simulink model "PMSM20180521"  (Simulink 7.9)
settings: Solver=FixedStepDiscrete  StartTime=0.0  StopTime=1  FixedStep=Auto  RelTol=1e-3
model workspace (MAT data in the model file):
  polePairs = 16
  encoderResolution = 4096
  indexOffset = 0
undefined symbols (not defined in the file or in its folder): Down, Up
libraries: idelinklib_common x37, simulink x13, c2833xlib x7, c280xlib x6, simulink_extras x2, idelinklib_ticcs x1, idelinklib_tgtpref x1
(part 1 of 3)
settings Model: Creator=ChenYu  LastModifiedBy=KING
settings DataIOCC: SaveOutput=off  SaveTime=off
settings OptimizationCC: OptimizeModelRefInitCode=on  LifeSpan=1
settings HardwareCC: ProdBitPerChar=16  ProdBitPerInt=16  ProdBitPerPointer=16  ProdLargestAtomicInteger=Integer  ProdIntDivRoundTo=Zero  ProdEndianess=LittleEndian  ProdWordSize=16  ProdHWDeviceType=Texas Instruments->C2000
settings RTWCC: SystemTargetFile=idelink_ert.tlc  GenerateMakefile=off  TemplateMakefile=none  Description=IDE Link ERT  ProcessScript=idelink_ert_make_rtw_hook
settings RTWCC: CustomInitializer=|
  | // Make sure the XINTF clock is enabled   cool
  | 	SysCtrlRegs.PCLKCR3.bit.XINTFENCLK = 1;
  | 
  | 	// Configure the GPIO for XINTF with a 16-bit data bus
  | 	// This function is in DSP2833x_Xintf.c
  | 	//InitXintf16Gpio();
  | 
  |     EALLOW;
  |     // All Zones---------------------------------
  |     // Timing for all zones based on XTIMCLK = SYSCLKOUT/2
  |     XintfRegs.XINTCNF2.bit.XTIMCLK = 1;
  |     // Buffer up to 3 writes
  |     XintfRegs.XINTCNF2.bit.WRBUFF = 3;
  |     // XCLKOUT is enabled
  |     XintfRegs.XINTCNF2.bit.CLKOFF = 0;
  |     // XCLKOUT = XTIMCLK/2
  |     XintfRegs.XINTCNF2.bit.CLKMODE = 1;
  | 
  |     // Zone 7------------------------------------
  |     // When using ready, ACTIVE must be 1 or greater
  |     // Lead must always be 1 or greater
  |     // Zone write timing
  |     XintfRegs.XTIMING7.bit.XWRLEAD = 3;//3*2*2*SYSCLKOUT
  |     XintfRegs.XTIMING7.bit.XWRACTIVE = 7; //(7+1)*2*2*SYSCLKOUT
  |     XintfRegs.XTIMING7.bit.XWRTRAIL = 3;
  |     // Zone read timing
  |     XintfRegs.XTIMING7.bit.XRDLEAD = 3;
  |     XintfRegs.XTIMING7.bit.XRDACTIVE = 7;
  |     XintfRegs.XTIMING7.bit.XRDTRAIL = 3;
  | 
  |     // double all Zone read/write lead/active/trail timing
  |     XintfRegs.XTIMING7.bit.X2TIMING = 1;
  | 
  |     // Zone will not sample XREADY signal
  |     XintfRegs.XTIMING7.bit.USEREADY = 0;
  |     XintfRegs.XTIMING7.bit.READYMODE = 0;
  | 
  |     // Size must be either:
  |     // 0,1 = x32 or
  |     // 1,1 = x16 other values are reserved
  |     XintfRegs.XTIMING7.bit.XSIZE = 3;
  | 
  |     EDIS;
  | 
  |    //Force a pipeline flush to ensure that the write to
  |    //the last register configured occurs before returning.
  |    asm(" RPT #7 || NOP");
settings CodeAppCC: IgnoreCustomStorageClasses=off
settings ERTFactory: TargetFcnLib=ansi_tfl_table_tmw.mat  CodeReplacementLibrary=ANSI_C  UtilityFuncGeneration=Auto  ERTMultiwordTypeDef=System defined  CodeExecutionProfiling=off  ERTMultiwordLength=256  MultiwordLength=2048  GenerateFullHeader=on  GenerateSampleERTMain=off  GenerateTestInterfaces=off  IsPILTarget=off  ModelReferenceCompliant=on  ParMdlRefBuildCompliant=off  CompOptLevelCompliant=off  ConcurrentExecutionCompliant=on  IncludeMdlTerminateFcn=on  GeneratePreprocessorConditionals=Disable all  CombineOutputUpdateFcns=on  CombineSignalStateStructs=off  SuppressErrorStatus=off  ERTFirstTimeCompliant=on  IncludeFileDelimiter=Auto  ERTCustomFileBanners=on  SupportAbsoluteTime=on  LogVarNameModifier=rt_  MatFileLogging=off  MultiInstanceERTCode=off  SupportNonFinite=on  SupportComplex=on  PurelyIntegerCode=off  SupportContinuousTime=off  SupportNonInlinedSFcns=off  SupportVariableSizeSignals=off  EnableShiftOperators=on  ParenthesesLevel=Nominal  PortableWordSizes=off  ModelStepFunctionPrototypeControlCompliant=on  CPPClassGenCompliant=off  AutosarCompliant=off  GRTInterface=off  GenerateErtSFunction=off  CreateSILPILBlock=None  CodeExecutionProfileVariable=executionProfile  CodeProfilingSaveOptions=SummaryOnly  GenerateASAP2=off  ExtMode=off  ExtModeTransport=0  ExtModeStaticAlloc=off  ExtModeStaticAllocSize=1000000  ExtModeTesting=off  ExtModeMexFile=TIC2000ExternalModeOpen  ExtModeIntrfLevel=Level2 - Open  InlinedParameterPlacement=Hierarchical  TargetOS=BareBoardExample  MultiInstanceErrorCode=Error  RateGroupingCode=on  RootIOFormat=Individual arguments  RTWCAPISignals=off  RTWCAPIParams=off  RTWCAPIStates=off  RTWCAPIRootIO=off  ERTSrcFileBannerTemplate=ert_code_template.cgt  ERTHdrFileBannerTemplate=ert_code_template.cgt  ERTDataSrcFileTemplate=ert_code_template.cgt  ERTDataHdrFileTemplate=ert_code_template.cgt  ERTCustomFileTemplate=example_file_process.tlc  CoverageDialogOpen=off  EnableDataOwnership=off  SignalDisplayLevel=10  ParamTuneLevel=10  GlobalDataDefinition=Auto  DataDefinitionFile=global.c  GlobalDataReference=Auto  ERTFilePackagingFormat=Modular  DataReferenceFile=global.h  PreserveExpressionOrder=off  PreserveIfCondition=off  ConvertIfToSwitch=off  PreserveExternInFcnDecls=on  SuppressUnreachableDefaultCases=off  EnableUserReplacementTypes=off  MemSecPackage=--- None ---  MemSecDataConstants=Default  MemSecDataIO=Default  MemSecDataInternal=Default  MemSecDataParameters=Default  MemSecFuncInitTerm=Default  MemSecFuncExecute=Default  MemSecFuncSharedUtil=Default  CodeProfilingInstrumentation=off  AdaptorName=Texas Instruments Code Composer Studio  exportIDEObj=on  ideObjName=IDE_Obj  oldideObjName=IDE_Obj  ideObjTimeout=10  oldideObjTimeout=10  ideObjBuildTimeout=1000  oldideObjBuildTimeout=1000  TargetPrefTimeStamp=01-Sep-2017 16:33:35  ProfileGenCode=on  profileBy=Tasks  ProfileNumSamples=100  InlineDSPBlks=off  projectOptions=Custom  debugCompilerOptions="-g -D\"_DEBUG\""  releaseCompilerOptions=-o2  getCompilerOptions=off  resetCompilerOptions=off  getLinkerOptions=off  resetLinkerOptions=off  systemStackSize=512  systemHeapSize=512  buildFormat=Project  buildAction=Build  overrunNotificationMethod=None  overrunNotificationFcn=myfunction  oldoverrunNotificationFcn=myfunction  configurePIL=off  configPILBlockAction=Create_PIL_block_build_and_download  DiagnosticActions=warning

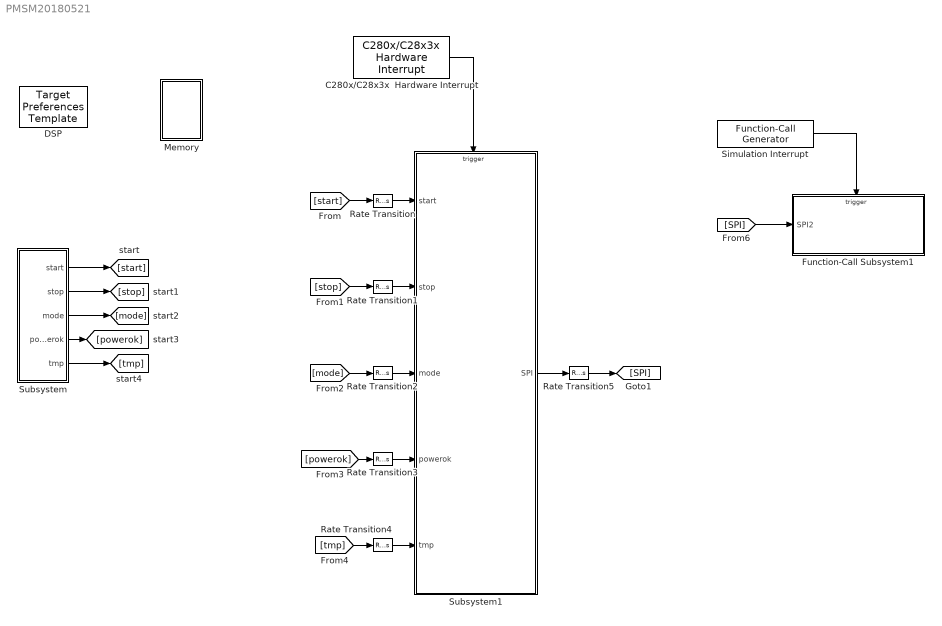
== system PMSM20180521 ==
  C280x/C28x3x  Hardware Interrupt : idelinklib_ticcs/C280x//C28x3x Hardware Interrupt  irqnumbers=[3]  pienumbers=[1]  irqpriorities=[30]  irqpreempts=[0]  showinput=off  dspchiptype=C280X
  DSP : idelinklib_tgtpref/Target Preferences Template  Tag=ccslinktgtpref  library=off
  Function-Call Subsystem1 : Subsystem  TreatAsAtomicUnit=on
  Memory : Subsystem
  Rate Transition{,1..5} (6 alike) : RateTransition  Integrity=off
  Simulation Interrupt : simulink/Ports & Subsystems/Function-Call Generator  sample_time=0.005  numberOfIterations=1
  Subsystem : Subsystem
  Subsystem1 : Subsystem
  wires:
  Subsystem/1(start) -> [start]
  Subsystem/2(stop) -> [stop]
  Subsystem/3(mode) -> [mode]
  Subsystem/4(powerok) -> [powerok]
  Subsystem/5(tmp) -> [tmp]
  [start] -> Rate Transition/1
  [stop] -> Rate Transition1/1
  [mode] -> Rate Transition2/1
  [powerok] -> Rate Transition3/1
  [tmp] -> Rate Transition4/1
  Rate Transition/1 -> Subsystem1/1(start)
  Rate Transition1/1 -> Subsystem1/2(stop)
  Rate Transition2/1 -> Subsystem1/3(mode)
  Rate Transition3/1 -> Subsystem1/4(powerok)
  C280x/C28x3x  Hardware Interrupt/1 -> Subsystem1/Trigger
  Rate Transition4/1 -> Subsystem1/5(tmp)
  [SPI] -> Function-Call Subsystem1/1(SPI2)
  Simulation Interrupt/1 -> Function-Call Subsystem1/Trigger
  Rate Transition5/1 -> [SPI]
  Subsystem1/1(SPI) -> Rate Transition5/1

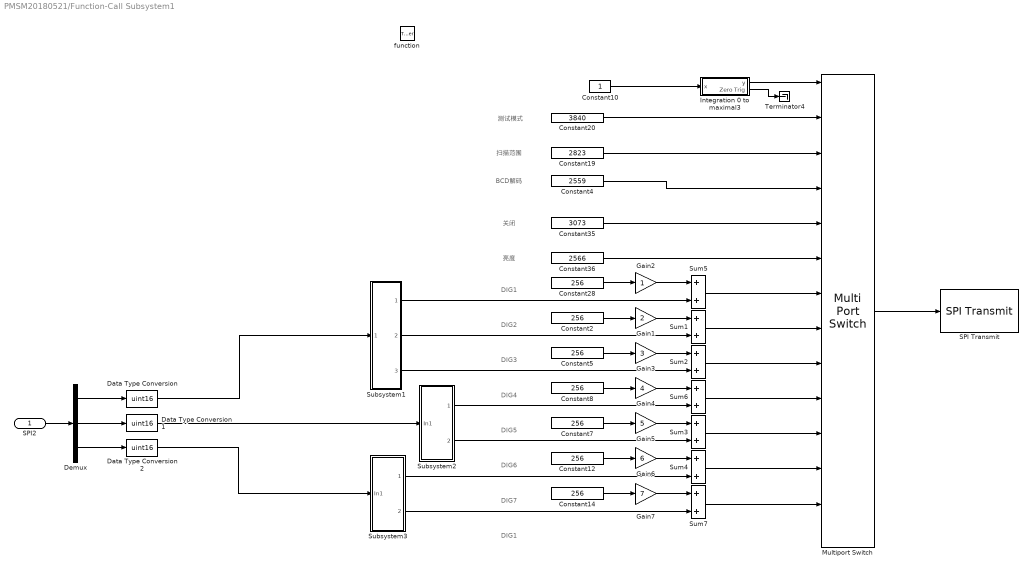
== system PMSM20180521/Function-Call Subsystem1 ==
  note: 扫描范围
  note: 测试模式
  note: BCD解码
  note: 关闭
  note: 亮度
  note: DIG1
  note: DIG2
  note: DIG3
  note: DIG4
  note: DIG5
  note: DIG6
  note: DIG7
  note: DIG1
  SPI2 : Inport
  function : TriggerPort  TriggerType=function-call
  Constant10 : Constant  OutDataTypeStr=uint16
  Constant{2,5,7..8,12,14,28} (7 alike) : Constant  Value=256  OutDataTypeStr=uint16
  Constant19 : Constant  Value=2823  OutDataTypeStr=uint16
  Constant20 : Constant  Value=3840  OutDataTypeStr=uint16
  Constant35 : Constant  Value=3073  OutDataTypeStr=uint16
  Constant36 : Constant  Value=2566  OutDataTypeStr=uint16
  Constant4 : Constant  Value=2559  OutDataTypeStr=uint16
  Data Type Conversion : DataTypeConversion  OutDataTypeStr=uint16
  Data Type Conversion1 : DataTypeConversion  OutDataTypeStr=uint16
  Data Type Conversion2 : DataTypeConversion  OutDataTypeStr=uint16
  Demux : Demux  Outputs=3
  Gain1 : Gain  Gain=2
  Gain2 : Gain
  Gain3 : Gain  Gain=3
  Gain4 : Gain  Gain=4
  Gain5 : Gain  Gain=5
  Gain6 : Gain  Gain=6
  Gain7 : Gain  Gain=7
  Integration 0 to maximal3 : Subsystem  mask{a=12}
      mask prompts: a "the maximal y"
  Multiport Switch : MultiPortSwitch  Inputs=12  DataPortForDefault=Additional data port  zeroidx=off  OutDataTypeStr=uint16
  SPI Transmit : c280xlib/SPI Transmit  selectModule=SPI_A  errFlag=off  enableBlocking=off  enableTxInt=off
  Subsystem1 : Subsystem
  Subsystem2 : Subsystem
  Subsystem3 : Subsystem
  Sum{1..7} (7 alike) : Sum
  Terminator4 : Terminator
  wires:
  Constant10/1 -> Integration 0 to maximal3/1(x)
  Constant19/1 -> Multiport Switch/3
  Constant20/1 -> Multiport Switch/2
  Integration 0 to maximal3/1(y) -> Multiport Switch/1
  Constant35/1 -> Multiport Switch/5
  Constant36/1 -> Multiport Switch/6
  Multiport Switch/1 -> SPI Transmit/1
  Constant28/1 -> Gain2/1
  Sum5/1 -> Multiport Switch/7
  Constant2/1 -> Gain1/1
  Sum1/1 -> Multiport Switch/8
  Constant5/1 -> Gain3/1
  Sum2/1 -> Multiport Switch/9
  Sum6/1 -> Multiport Switch/10
  Subsystem2/1(Out2) -> Sum6/2
  Constant7/1 -> Gain5/1
  Sum3/1 -> Multiport Switch/11
  Subsystem2/2(Out3) -> Sum3/2
  Constant12/1 -> Gain6/1
  Sum4/1 -> Multiport Switch/12
  Subsystem3/1(Out2) -> Sum4/2
  Constant14/1 -> Gain7/1
  Sum7/1 -> Multiport Switch/13
  Gain2/1 -> Sum5/1
  Constant8/1 -> Gain4/1
  Gain1/1 -> Sum1/1
  Gain3/1 -> Sum2/1
  Gain4/1 -> Sum6/1
  Gain5/1 -> Sum3/1
  Gain6/1 -> Sum4/1
  Subsystem3/2(Out3) -> Sum7/2
  Gain7/1 -> Sum7/1
  Constant4/1 -> Multiport Switch/4
  Subsystem1/1(Out1) -> Sum5/2
  Subsystem1/2(Out2) -> Sum1/2
  Subsystem1/3(Out3) -> Sum2/2
  Demux/1 -> Data Type Conversion/1
  Demux/2 -> Data Type Conversion1/1
  Demux/3 -> Data Type Conversion2/1
  SPI2/1 -> Demux/1
  Data Type Conversion/1 -> Subsystem1/1(In1)
  Data Type Conversion1/1 -> Subsystem2/1(In1)
  Data Type Conversion2/1 -> Subsystem3/1(In1)
  Integration 0 to maximal3/2(Zero Trig) -> Terminator4/1

== system PMSM20180521/Memory ==
  Memory Allocate : idelinklib_common/Memory Allocate  variableName=p1  alignThisVariable=off  memoryAlignmentBoundary=4  dataType=int16  specifyQualifier=off  typeQualifier=volatile  dataDimension=1  specifyMemorySection=off  memorySection=mySEC1  bindMemorySection=off  sectionStartAddress=hex2dec('8000')  initializeMemory=on  initialValue=0
  Memory Allocate1 : idelinklib_common/Memory Allocate  variableName=p2  alignThisVariable=off  memoryAlignmentBoundary=4  dataType=int16  specifyQualifier=off  typeQualifier=volatile  dataDimension=1  specifyMemorySection=off  memorySection=mySEC1  bindMemorySection=off  sectionStartAddress=hex2dec('8000')  initializeMemory=on  initialValue=0
  Memory Allocate10 : idelinklib_common/Memory Allocate  variableName=p11  alignThisVariable=off  memoryAlignmentBoundary=4  dataType=int16  specifyQualifier=off  typeQualifier=volatile  dataDimension=1  specifyMemorySection=off  memorySection=mySEC1  bindMemorySection=off  sectionStartAddress=hex2dec('8000')  initializeMemory=on  initialValue=0
  Memory Allocate11 : idelinklib_common/Memory Allocate  variableName=data1  alignThisVariable=off  memoryAlignmentBoundary=4  dataType=int16  specifyQualifier=off  typeQualifier=volatile  dataDimension=1  specifyMemorySection=off  memorySection=mySEC1  bindMemorySection=off  sectionStartAddress=hex2dec('8000')  initializeMemory=on  initialValue=0
  Memory Allocate12 : idelinklib_common/Memory Allocate  variableName=data2  alignThisVariable=off  memoryAlignmentBoundary=4  dataType=int16  specifyQualifier=off  typeQualifier=volatile  dataDimension=1  specifyMemorySection=off  memorySection=mySEC1  bindMemorySection=off  sectionStartAddress=hex2dec('8000')  initializeMemory=on  initialValue=0
  Memory Allocate13 : idelinklib_common/Memory Allocate  variableName=data3  alignThisVariable=off  memoryAlignmentBoundary=4  dataType=int16  specifyQualifier=off  typeQualifier=volatile  dataDimension=1  specifyMemorySection=off  memorySection=mySEC1  bindMemorySection=off  sectionStartAddress=hex2dec('8000')  initializeMemory=on  initialValue=0
  Memory Allocate14 : idelinklib_common/Memory Allocate  variableName=data4  alignThisVariable=off  memoryAlignmentBoundary=4  dataType=int16  specifyQualifier=off  typeQualifier=volatile  dataDimension=1  specifyMemorySection=off  memorySection=mySEC1  bindMemorySection=off  sectionStartAddress=hex2dec('8000')  initializeMemory=on  initialValue=0
  Memory Allocate15 : idelinklib_common/Memory Allocate  variableName=data5  alignThisVariable=off  memoryAlignmentBoundary=4  dataType=int16  specifyQualifier=off  typeQualifier=volatile  dataDimension=1  specifyMemorySection=off  memorySection=mySEC1  bindMemorySection=off  sectionStartAddress=hex2dec('8000')  initializeMemory=on  initialValue=0
  Memory Allocate16 : idelinklib_common/Memory Allocate  variableName=data6  alignThisVariable=off  memoryAlignmentBoundary=4  dataType=int16  specifyQualifier=off  typeQualifier=volatile  dataDimension=1  specifyMemorySection=off  memorySection=mySEC1  bindMemorySection=off  sectionStartAddress=hex2dec('8000')  initializeMemory=on  initialValue=0
  Memory Allocate17 : idelinklib_common/Memory Allocate  variableName=data7  alignThisVariable=off  memoryAlignmentBoundary=4  dataType=int16  specifyQualifier=off  typeQualifier=volatile  dataDimension=1  specifyMemorySection=off  memorySection=mySEC1  bindMemorySection=off  sectionStartAddress=hex2dec('8000')  initializeMemory=on  initialValue=0
  Memory Allocate18 : idelinklib_common/Memory Allocate  variableName=data8  alignThisVariable=off  memoryAlignmentBoundary=4  dataType=int16  specifyQualifier=off  typeQualifier=volatile  dataDimension=1  specifyMemorySection=off  memorySection=mySEC1  bindMemorySection=off  sectionStartAddress=hex2dec('8000')  initializeMemory=on  initialValue=0
  Memory Allocate19 : idelinklib_common/Memory Allocate  variableName=data9  alignThisVariable=off  memoryAlignmentBoundary=4  dataType=int16  specifyQualifier=off  typeQualifier=volatile  dataDimension=1  specifyMemorySection=off  memorySection=mySEC1  bindMemorySection=off  sectionStartAddress=hex2dec('8000')  initializeMemory=on  initialValue=0
  Memory Allocate2 : idelinklib_common/Memory Allocate  variableName=p3  alignThisVariable=off  memoryAlignmentBoundary=4  dataType=int16  specifyQualifier=off  typeQualifier=volatile  dataDimension=1  specifyMemorySection=off  memorySection=mySEC1  bindMemorySection=off  sectionStartAddress=hex2dec('8000')  initializeMemory=on  initialValue=0
  Memory Allocate20 : idelinklib_common/Memory Allocate  variableName=data10  alignThisVariable=off  memoryAlignmentBoundary=4  dataType=int16  specifyQualifier=off  typeQualifier=volatile  dataDimension=1  specifyMemorySection=off  memorySection=mySEC1  bindMemorySection=off  sectionStartAddress=hex2dec('8000')  initializeMemory=on  initialValue=0
  Memory Allocate21 : idelinklib_common/Memory Allocate  variableName=data11  alignThisVariable=off  memoryAlignmentBoundary=4  dataType=int16  specifyQualifier=off  typeQualifier=volatile  dataDimension=1  specifyMemorySection=off  memorySection=mySEC1  bindMemorySection=off  sectionStartAddress=hex2dec('8000')  initializeMemory=on  initialValue=0
  Memory Allocate22 : idelinklib_common/Memory Allocate  variableName=data12  alignThisVariable=off  memoryAlignmentBoundary=4  dataType=int16  specifyQualifier=off  typeQualifier=volatile  dataDimension=1  specifyMemorySection=off  memorySection=mySEC1  bindMemorySection=off  sectionStartAddress=hex2dec('8000')  initializeMemory=on  initialValue=0
  Memory Allocate3 : idelinklib_common/Memory Allocate  variableName=p4  alignThisVariable=off  memoryAlignmentBoundary=4  dataType=int16  specifyQualifier=off  typeQualifier=volatile  dataDimension=1  specifyMemorySection=off  memorySection=mySEC1  bindMemorySection=off  sectionStartAddress=hex2dec('8000')  initializeMemory=on  initialValue=0
  Memory Allocate4 : idelinklib_common/Memory Allocate  variableName=p5  alignThisVariable=off  memoryAlignmentBoundary=4  dataType=int16  specifyQualifier=off  typeQualifier=volatile  dataDimension=1  specifyMemorySection=off  memorySection=mySEC1  bindMemorySection=off  sectionStartAddress=hex2dec('8000')  initializeMemory=on  initialValue=0
  Memory Allocate5 : idelinklib_common/Memory Allocate  variableName=p6  alignThisVariable=off  memoryAlignmentBoundary=4  dataType=int16  specifyQualifier=off  typeQualifier=volatile  dataDimension=1  specifyMemorySection=off  memorySection=mySEC1  bindMemorySection=off  sectionStartAddress=hex2dec('8000')  initializeMemory=on  initialValue=0
  Memory Allocate6 : idelinklib_common/Memory Allocate  variableName=p7  alignThisVariable=off  memoryAlignmentBoundary=4  dataType=int16  specifyQualifier=off  typeQualifier=volatile  dataDimension=1  specifyMemorySection=off  memorySection=mySEC1  bindMemorySection=off  sectionStartAddress=hex2dec('8000')  initializeMemory=on  initialValue=0
  Memory Allocate7 : idelinklib_common/Memory Allocate  variableName=p8  alignThisVariable=off  memoryAlignmentBoundary=4  dataType=int16  specifyQualifier=off  typeQualifier=volatile  dataDimension=1  specifyMemorySection=off  memorySection=mySEC1  bindMemorySection=off  sectionStartAddress=hex2dec('8000')  initializeMemory=on  initialValue=0
  Memory Allocate8 : idelinklib_common/Memory Allocate  variableName=p9  alignThisVariable=off  memoryAlignmentBoundary=4  dataType=int16  specifyQualifier=off  typeQualifier=volatile  dataDimension=1  specifyMemorySection=off  memorySection=mySEC1  bindMemorySection=off  sectionStartAddress=hex2dec('8000')  initializeMemory=on  initialValue=0
  Memory Allocate9 : idelinklib_common/Memory Allocate  variableName=p10  alignThisVariable=off  memoryAlignmentBoundary=4  dataType=int16  specifyQualifier=off  typeQualifier=volatile  dataDimension=1  specifyMemorySection=off  memorySection=mySEC1  bindMemorySection=off  sectionStartAddress=hex2dec('8000')  initializeMemory=on  initialValue=0

== system PMSM20180521/Subsystem ==
  MODE : c2833xlib/Digital Input  GPIO_Number=GPIO40~GPIO47  GPIO_Bit0=on  GPIO_Bit1=off  GPIO_Bit2=off  GPIO_Bit3=off  GPIO_Bit4=off  GPIO_Bit5=off  GPIO_Bit6=off  GPIO_Bit7=off  sampleTime=-1  dataType=boolean  GPIO_Bit0_Qualification=Sync to SYSCLKOUT  GPIO_Bit1_Qualification=Sync to SYSCLKOUT  GPIO_Bit2_Qualification=Sync to SYSCLKOUT  GPIO_Bit3_Qualification=Sync to SYSCLKOUT  GPIO_Bit4_Qualification=Sync to SYSCLKOUT  GPIO_Bit5_Qualification=Sync to SYSCLKOUT  GPIO_Bit6_Qualification=Sync to SYSCLKOUT  GPIO_Bit7_Qualification=Sync to SYSCLKOUT  Qualification_Period=-1
  MODE1 : c2833xlib/Digital Input  GPIO_Number=GPIO32~GPIO39  GPIO_Bit0=off  GPIO_Bit1=on  GPIO_Bit2=off  GPIO_Bit3=off  GPIO_Bit4=off  GPIO_Bit5=off  GPIO_Bit6=off  GPIO_Bit7=off  sampleTime=-1  dataType=boolean  GPIO_Bit0_Qualification=Sync to SYSCLKOUT  GPIO_Bit1_Qualification=Sync to SYSCLKOUT  GPIO_Bit2_Qualification=Sync to SYSCLKOUT  GPIO_Bit3_Qualification=Sync to SYSCLKOUT  GPIO_Bit4_Qualification=Sync to SYSCLKOUT  GPIO_Bit5_Qualification=Sync to SYSCLKOUT  GPIO_Bit6_Qualification=Sync to SYSCLKOUT  GPIO_Bit7_Qualification=Sync to SYSCLKOUT  Qualification_Period=-1
  MODE2 : c2833xlib/Digital Input  GPIO_Number=GPIO32~GPIO39  GPIO_Bit0=on  GPIO_Bit1=off  GPIO_Bit2=off  GPIO_Bit3=off  GPIO_Bit4=off  GPIO_Bit5=off  GPIO_Bit6=off  GPIO_Bit7=off  sampleTime=-1  dataType=boolean  GPIO_Bit0_Qualification=Sync to SYSCLKOUT  GPIO_Bit1_Qualification=Sync to SYSCLKOUT  GPIO_Bit2_Qualification=Sync to SYSCLKOUT  GPIO_Bit3_Qualification=Sync to SYSCLKOUT  GPIO_Bit4_Qualification=Sync to SYSCLKOUT  GPIO_Bit5_Qualification=Sync to SYSCLKOUT  GPIO_Bit6_Qualification=Sync to SYSCLKOUT  GPIO_Bit7_Qualification=Sync to SYSCLKOUT  Qualification_Period=-1
  PB-OFF : c2833xlib/Digital Input  GPIO_Number=GPIO32~GPIO39  GPIO_Bit0=off  GPIO_Bit1=off  GPIO_Bit2=on  GPIO_Bit3=off  GPIO_Bit4=off  GPIO_Bit5=off  GPIO_Bit6=off  GPIO_Bit7=off  sampleTime=-1  dataType=boolean  GPIO_Bit0_Qualification=Sync to SYSCLKOUT  GPIO_Bit1_Qualification=Sync to SYSCLKOUT  GPIO_Bit2_Qualification=Sync to SYSCLKOUT  GPIO_Bit3_Qualification=Sync to SYSCLKOUT  GPIO_Bit4_Qualification=Sync to SYSCLKOUT  GPIO_Bit5_Qualification=Sync to SYSCLKOUT  GPIO_Bit6_Qualification=Sync to SYSCLKOUT  GPIO_Bit7_Qualification=Sync to SYSCLKOUT  Qualification_Period=-1
  PB-ON : c2833xlib/Digital Input  GPIO_Number=GPIO32~GPIO39  GPIO_Bit0=off  GPIO_Bit1=off  GPIO_Bit2=off  GPIO_Bit3=on  GPIO_Bit4=off  GPIO_Bit5=off  GPIO_Bit6=off  GPIO_Bit7=off  sampleTime=-1  dataType=boolean  GPIO_Bit0_Qualification=Sync to SYSCLKOUT  GPIO_Bit1_Qualification=Sync to SYSCLKOUT  GPIO_Bit2_Qualification=Sync to SYSCLKOUT  GPIO_Bit3_Qualification=Sync to SYSCLKOUT  GPIO_Bit4_Qualification=Sync to SYSCLKOUT  GPIO_Bit5_Qualification=Sync to SYSCLKOUT  GPIO_Bit6_Qualification=Sync to SYSCLKOUT  GPIO_Bit7_Qualification=Sync to SYSCLKOUT  Qualification_Period=-1
  start : Outport
  stop : Outport  Port=2
  mode : Outport  Port=3
  powerok : Outport  Port=4
  tmp : Outport  Port=5
  wires:
  PB-ON/1 -> start/1
  PB-OFF/1 -> stop/1
  MODE/1 -> mode/1
  MODE1/1 -> powerok/1
  MODE2/1 -> tmp/1

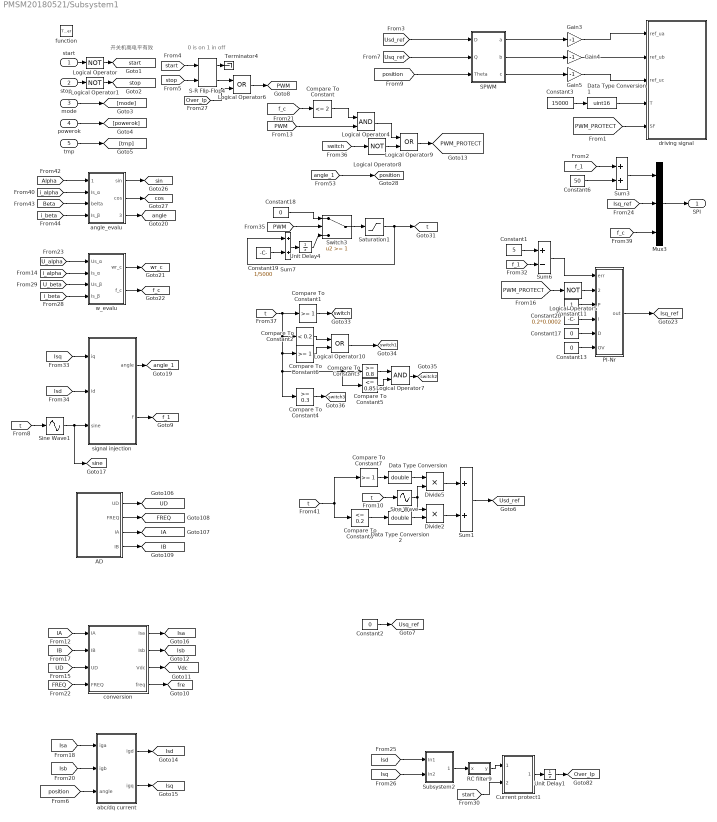
== system PMSM20180521/Subsystem1 ==
  note: 开关机高电平有效
  note: 0 is on 1 in off
  start : Inport
  stop : Inport  Port=2
  mode : Inport  Port=3
  powerok : Inport  Port=4
  tmp : Inport  Port=5
  function : TriggerPort  TriggerType=function-call
  AD : Subsystem
  Compare To Constant : simulink/Logic and Bit Operations/Compare To Constant  relop=<=  const=2  OutDataTypeStr=boolean
  Compare To Constant1 : simulink/Logic and Bit Operations/Compare To Constant  relop=>=  const=1  OutDataTypeStr=boolean
  Compare To Constant2 : simulink/Logic and Bit Operations/Compare To Constant  relop=<  const=0.2  OutDataTypeStr=boolean
  Compare To Constant3 : simulink/Logic and Bit Operations/Compare To Constant  relop=>=  const=0.8  OutDataTypeStr=boolean
  Compare To Constant4 : simulink/Logic and Bit Operations/Compare To Constant  relop=>=  const=0.3  OutDataTypeStr=boolean
  Compare To Constant5 : simulink/Logic and Bit Operations/Compare To Constant  relop=<=  const=0.85  OutDataTypeStr=boolean
  Compare To Constant6 : simulink/Logic and Bit Operations/Compare To Constant  relop=>=  const=1  OutDataTypeStr=boolean
  Compare To Constant7 : simulink/Logic and Bit Operations/Compare To Constant  relop=>=  const=1  OutDataTypeStr=boolean
  Compare To Constant8 : simulink/Logic and Bit Operations/Compare To Constant  relop=<=  const=0.2  OutDataTypeStr=boolean
  Constant1 : Constant  Value=5  OutDataTypeStr=double
  Constant11 : Constant  OutDataTypeStr=double
  Constant{2,13,17..18} (4 alike) : Constant  Value=0  OutDataTypeStr=double
  Constant19 : Constant  Value=1/5000  OutDataTypeStr=double
  Constant20 : Constant  Value=0.2*0.0002  OutDataTypeStr=double
  Constant3 : Constant  Value=15000  OutDataTypeStr=int16
  Constant6 : Constant  Value=50  OutDataTypeStr=double
  Current protect1 : Subsystem
  Data Type Conversion : DataTypeConversion  OutDataTypeStr=double
  Data Type Conversion1 : DataTypeConversion  OutDataTypeStr=uint16
  Data Type Conversion2 : DataTypeConversion  OutDataTypeStr=double
  Divide2 : Product  Inputs=**
  Divide5 : Product  Inputs=**
  Gain3 : Gain  Gain=-1
  Gain4 : Gain  Gain=-1
  Gain5 : Gain  Gain=-1
  Logical Operator{,1,5,8} (4 alike) : Logic  Operator=NOT  AllPortsSameDT=off  OutDataTypeStr=boolean
  Logical Operator10 : Logic  Operator=OR  AllPortsSameDT=off  OutDataTypeStr=boolean
  Logical Operator4 : Logic  AllPortsSameDT=off  OutDataTypeStr=boolean
  Logical Operator6 : Logic  Operator=OR  AllPortsSameDT=off  OutDataTypeStr=boolean
  Logical Operator7 : Logic  AllPortsSameDT=off  OutDataTypeStr=boolean
  Logical Operator9 : Logic  Operator=OR  AllPortsSameDT=off  OutDataTypeStr=boolean
  Mux3 : Mux  Inputs=3
  PI-Nr : Subsystem  mask{ermax=15, ermin=-15, max=19, min=0}
      mask prompts: ermax "Err max limit"; ermin "Err min limit"; max "Output max limit"; min "Output min limit"
  RC filter9 : Subsystem  mask{a=0.5}
      mask prompts: a "Time Constant"
  S-R Flip-Flop4 : simulink_extras/Flip Flops/S-R Flip-Flop  initial_condition=0
  SPWM : Subsystem
  Saturation1 : Saturate  UpperLimit=40  LowerLimit=0  LinearizeAsGain=off  ZeroCross=off  OutDataTypeStr=double
  Sine Wave : Sin  TimeSource=Use external signal  Amplitude=0.05  Frequency=2*pi*400  Phase=0.5*pi  VectorParams1D=off
  Sine Wave1 : Sin  TimeSource=Use external signal  Frequency=2*pi*400  VectorParams1D=off
  Subsystem2 : Subsystem
  Sum1 : Sum  Inputs=2
  Sum3 : Sum  Inputs=2
  Sum6 : Sum  Inputs=+-
  Sum7 : Sum
  Switch3 : Switch  Threshold=1
  Terminator4 : Terminator
  Unit Delay1 : UnitDelay  SampleTime=-1
  Unit Delay4 : UnitDelay  SampleTime=-1
  abc/dq current : Subsystem
  angle_evalu : Subsystem
  conversion : Subsystem
  driving signal : Subsystem
  signal injection : Subsystem
  w_evalu : Subsystem
  SPI : Outport
  tag scope: FREQ=global, IA=global, IB=global, Isa=global, Isb=global, Isd=global, Isq=global, Isq_ref=global, Over_Ip=global, PWM=global, PWM_PROTECT=global, UD=global, Usd_ref=global, Usq_ref=global, Vdc=global, angle=global, angle_1=global, cos=global, f_1=global, f_c=global, fre=global, position=global, sin=global, sine=global, start=global, stop=global, switch1=global, switch2=global, switch3=global, switch=global, t=global, wr_c=global
  wires:
  Constant3/1 -> Data Type Conversion1/1
  start/1 -> Logical Operator/1
  stop/1 -> Logical Operator1/1
  mode/1 -> [mode]
  powerok/1 -> [powerok]
  tmp/1 -> [tmp]
  Logical Operator/1 -> [start]
  Logical Operator1/1 -> [stop]
  [start] -> S-R Flip-Flop4/1
  [stop] -> S-R Flip-Flop4/2
  S-R Flip-Flop4/1 -> Terminator4/1
  Data Type Conversion1/1 -> driving signal/4(T)
  [PWM_PROTECT] -> driving signal/5(SF)
  [Usd_ref] -> SPWM/1(D)
  [Usq_ref] -> SPWM/2(Q)
  [position] -> SPWM/3(Theta)
  [f_c] -> Compare To Constant/1
  [PWM] -> Logical Operator4/2
  Compare To Constant/1 -> Logical Operator4/1
  SPWM/1(a) -> Gain3/1
  Gain4/1 -> driving signal/2(ref_ub)
  Gain3/1 -> driving signal/1(ref_ua)
  Gain5/1 -> driving signal/3(ref_uc)
  SPWM/2(b) -> Gain4/1
  SPWM/3(c) -> Gain5/1
  AD/1(UD) -> [UD]
  AD/4(IB) -> [IB]
  AD/3(IA) -> [IA]
  AD/2(FREQ) -> [FREQ]
  conversion/1(Isa) -> [Isa]
  conversion/2(Isb) -> [Isb]
  [IB] -> conversion/2(IB)
  [IA] -> conversion/1(IA)
  [UD] -> conversion/3(UD)
  conversion/3(Vdc) -> [Vdc]
  [Isa] -> abc/dq current/1(iga)
  [Isb] -> abc/dq current/2(igb)
  [position] -> abc/dq current/3(angle)
  abc/dq current/1(igd) -> [Isd]
  abc/dq current/2(igq) -> [Isq]
  Constant2/1 -> [Usq_ref]
  [FREQ] -> conversion/4(FREQ)
  conversion/4(freq) -> [fre]
  [Isd] -> Subsystem2/1(In1)
  [Isq] -> Subsystem2/2(In2)
  RC filter9/1(y) -> Current protect1/1(igdin)
  Subsystem2/1(Out1) -> RC filter9/1(x)
  [start] -> Current protect1/2(reset)
  Unit Delay1/1 -> [Over_Ip]
  Current protect1/1(Software_I) -> Unit Delay1/1
  [Over_Ip] -> Logical Operator6/2
  S-R Flip-Flop4/2 -> Logical Operator6/1
  Logical Operator6/1 -> [PWM]
  Mux3/1 -> SPI/1
  [Alpha] -> angle_evalu/1(alpha)
  [Beta] -> angle_evalu/3(belta)
  [i_beta] -> angle_evalu/4(Is_β)
  [i_alpha] -> angle_evalu/2(Is_α)
  angle_evalu/1(sin) -> [sin]
  angle_evalu/2(cos) -> [cos]
  angle_evalu/3(angle_c) -> [angle]
  [f_c] -> Mux3/3
  [f_1] -> Sum6/2
  Sum6/1 -> PI-Nr/1(err)
  [PWM_PROTECT] -> Logical Operator5/1
  Constant13/1 -> PI-Nr/6(OV)
  Constant17/1 -> PI-Nr/5(D)
  Constant20/1 -> PI-Nr/4(I)
  Constant11/1 -> PI-Nr/3(P)
  Logical Operator5/1 -> PI-Nr/2(reset)
  PI-Nr/1(out) -> [Isq_ref]
  [Isq] -> signal injection/1(iq)
  Sine Wave1/1 -> signal injection/3(sine), [sine]
  signal injection/1(angle) -> [angle_1]
  signal injection/2(f) -> [f_1]
  [i_alpha] -> w_evalu/2(Is_α)
  [U_alpha] -> w_evalu/1(Us_α)
  [i_beta] -> w_evalu/4(Is_β)
  [U_beta] -> w_evalu/3(Us_β)
  w_evalu/1(wr_c) -> [wr_c]
  w_evalu/2(f_c) -> [f_c]
  [angle_1] -> [position]
  [Isq_ref] -> Mux3/2
  Constant1/1 -> Sum6/1
  [f_1] -> Sum3/1
  Sum3/1 -> Mux3/1
  Constant6/1 -> Sum3/2
  [Isd] -> signal injection/2(id)
  Sine Wave/1 -> Divide2/1, Divide5/2
  Data Type Conversion2/1 -> Divide2/2
  Sum1/1 -> [Usd_ref]
  Logical Operator8/1 -> Logical Operator9/2
  Logical Operator4/1 -> Logical Operator9/1
  Logical Operator9/1 -> [PWM_PROTECT]
  Data Type Conversion/1 -> Divide5/1
  Divide2/1 -> Sum1/2
  Divide5/1 -> Sum1/1
  [switch] -> Logical Operator8/1
  Constant18/1 -> Switch3/1
  [PWM] -> Switch3/2
  Constant19/1 -> Sum7/2
  Sum7/1 -> Unit Delay4/1
  Unit Delay4/1 -> Switch3/3
  Switch3/1 -> Saturation1/1
  Saturation1/1 -> [t], Sum7/1
  [t] -> Compare To Constant1/1, Compare To Constant2/1, Compare To Constant4/1, Compare To Constant3/1, Compare To Constant5/1, Compare To Constant6/1
  Compare To Constant1/1 -> [switch]
  Compare To Constant4/1 -> [switch3]
  Compare To Constant3/1 -> Logical Operator7/1
  Logical Operator7/1 -> [switch2]
  Compare To Constant5/1 -> Logical Operator7/2
  Logical Operator10/1 -> [switch1]
  Compare To Constant2/1 -> Logical Operator10/1
  Compare To Constant6/1 -> Logical Operator10/2
  Compare To Constant7/1 -> Data Type Conversion/1
  [t] -> Compare To Constant8/1, Compare To Constant7/1
  Compare To Constant8/1 -> Data Type Conversion2/1
  [t] -> Sine Wave1/1
  [t] -> Sine Wave/1

== system PMSM20180521/Function-Call Subsystem1/Integration 0 to maximal3 ==
  x : Inport
  3 : Constant  Value=a  OutDataTypeStr=fixdt(1,32,16)
  Relational Operator1 : RelationalOperator  Operator=<=
  Sum1 : Sum  Inputs=+-
  Sum2 : Sum
  Switch2 : Switch  Criteria=u2 > Threshold  SaturateOnIntegerOverflow=on  InputSameDT=on
  Unit Delay1 : UnitDelay  SampleTime=-1
  y : Outport
  Zero Trig : Outport  Port=2
  wires:
  x/1 -> Sum2/2
  Sum1/1 -> Switch2/3
  Switch2/1 -> y/1, Unit Delay1/1
  Relational Operator1/1 -> Zero Trig/1, Switch2/2
  3/1 -> Sum1/2, Relational Operator1/2
  Sum2/1 -> Sum1/1, Relational Operator1/1, Switch2/1
  Unit Delay1/1 -> Sum2/1

== system PMSM20180521/Function-Call Subsystem1/Subsystem1 ==
  In1 : Inport
  求个位 : Subsystem
  求十位 : Subsystem
  求百位 : Subsystem
  Out1 : Outport
  Out2 : Outport  Port=2
  Out3 : Outport  Port=3
  wires:
  In1/1 -> 求百位/1(In1), 求十位/2(In2), 求个位/1(In1)
  求个位/1(Out1) -> Out3/1
  求百位/1(Out1) -> Out1/1, 求十位/1(In1), 求个位/2(In2)
  求十位/1(Out1) -> Out2/1, 求个位/3(In3)

== system PMSM20180521/Function-Call Subsystem1/Subsystem2 ==
  In1 : Inport
  求个位 : Subsystem
  求十位 : Subsystem
  求百位 : Subsystem
  Out2 : Outport
  Out3 : Outport  Port=2
  wires:
  求十位/1(Out1) -> 求个位/3(In3), Out2/1
  求百位/1(Out1) -> 求个位/2(In2), 求十位/1(In1)
  求个位/1(Out1) -> Out3/1
  In1/1 -> 求个位/1(In1), 求十位/2(In2), 求百位/1(In1)

== system PMSM20180521/Function-Call Subsystem1/Subsystem3 ==
  In1 : Inport
  求个位 : Subsystem
  求十位 : Subsystem
  求百位 : Subsystem
  Out2 : Outport
  Out3 : Outport  Port=2
  wires:
  In1/1 -> 求百位/1(In1), 求十位/2(In2), 求个位/1(In1)
  求个位/1(Out1) -> Out3/1
  求百位/1(Out1) -> 求十位/1(In1), 求个位/2(In2)
  求十位/1(Out1) -> Out2/1, 求个位/3(In3)

== system PMSM20180521/Subsystem1/AD ==
  Start Conversion : Subsystem  Priority=1
  Stop Conversion : Subsystem  Priority=3
  read AD : Subsystem
  UD : Outport
  FREQ : Outport  Port=2
  IA : Outport  Port=3
  IB : Outport  Port=4
  wires:
  read AD/1(UD) -> UD/1
  read AD/2(UOUT) -> [UOUT]
  read AD/3(UOUT1) -> [UOUT1]
  read AD/4(FREQ) -> FREQ/1
  read AD/5(IA) -> IA/1
  read AD/6(IB) -> IB/1

== system PMSM20180521/Subsystem1/Current protect1 ==
  igdin : Inport
  reset : Inport  Port=2
  Constant25 : Constant  Value=0  OutDataTypeStr=boolean
  Constant26 : Constant  OutDataTypeStr=boolean
  S-R Flip-Flop1 : simulink_extras/Flip Flops/S-R Flip-Flop  initial_condition=0
  Switch9 : Switch  Criteria=u2 > Threshold  Threshold=120  SaturateOnIntegerOverflow=on  InputSameDT=on
  Terminator : Terminator
  Software_I : Outport
  wires:
  igdin/1 -> Switch9/2
  S-R Flip-Flop1/1 -> Software_I/1
  Constant25/1 -> Switch9/3
  Constant26/1 -> Switch9/1
  S-R Flip-Flop1/2 -> Terminator/1
  Switch9/1 -> S-R Flip-Flop1/1
  reset/1 -> S-R Flip-Flop1/2

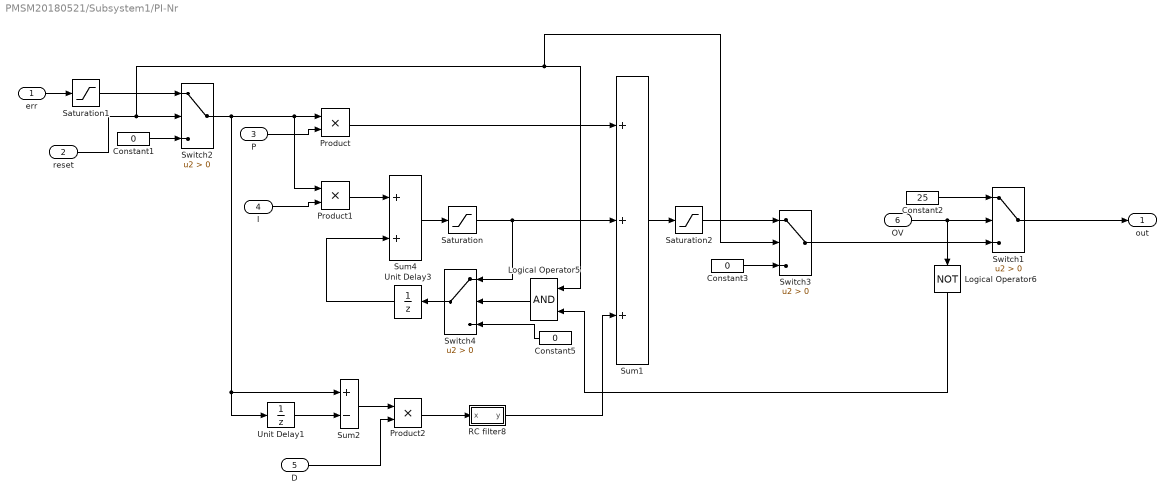
== system PMSM20180521/Subsystem1/PI-Nr ==
  err : Inport
  reset : Inport  Port=2
  P : Inport  Port=3
  I : Inport  Port=4
  D : Inport  Port=5
  OV : Inport  Port=6
  Constant1 : Constant  Value=0  OutDataTypeStr=Inherit: Inherit via back propagation
  Constant2 : Constant  Value=25  OutDataTypeStr=Inherit: Inherit via back propagation
  Constant3 : Constant  Value=0  OutDataTypeStr=Inherit: Inherit via back propagation
  Constant5 : Constant  Value=0  OutDataTypeStr=Inherit: Inherit via back propagation
  Logical Operator5 : Logic  AllPortsSameDT=off  OutDataTypeStr=boolean
  Logical Operator6 : Logic  Operator=NOT  AllPortsSameDT=off  OutDataTypeStr=boolean
  Product : Product  RndMeth=Zero
  Product1 : Product  RndMeth=Zero
  Product2 : Product  RndMeth=Zero
  RC filter8 : Subsystem  mask{a=0.4}
      mask prompts: a "Time Constant"
  Saturation : Saturate  UpperLimit=max  LowerLimit=min  LinearizeAsGain=off  ZeroCross=off  OutDataTypeStr=double
  Saturation1 : Saturate  UpperLimit=ermax  LowerLimit=ermin  LinearizeAsGain=off  ZeroCross=off  OutDataTypeStr=double
  Saturation2 : Saturate  UpperLimit=max  LowerLimit=min  LinearizeAsGain=off  ZeroCross=off  OutDataTypeStr=double
  Sum1 : Sum  Inputs=+++
  Sum2 : Sum  Inputs=+-
  Sum4 : Sum
  Switch{1..4} (4 alike) : Switch  Criteria=u2 > Threshold  SaturateOnIntegerOverflow=on  InputSameDT=on
  Unit Delay1 : UnitDelay  SampleTime=-1
  Unit Delay3 : UnitDelay  SampleTime=-1
  out : Outport
  wires:
  Logical Operator6/1 -> Logical Operator5/2
  Logical Operator5/1 -> Switch4/2
  RC filter8/1(y) -> Sum1/3
  Constant3/1 -> Switch3/3
  Switch3/1 -> Switch1/3
  Saturation2/1 -> Switch3/1
  Switch1/1 -> out/1
  OV/1 -> Logical Operator6/1, Switch1/2
  Constant2/1 -> Switch1/1
  Sum1/1 -> Saturation2/1
  Product2/1 -> RC filter8/1(x)
  Unit Delay1/1 -> Sum2/2
  D/1 -> Product2/2
  Sum2/1 -> Product2/1
  Switch4/1 -> Unit Delay3/1
  Unit Delay3/1 -> Sum4/2
  Saturation/1 -> Switch4/1, Sum1/2
  Sum4/1 -> Saturation/1
  Product1/1 -> Sum4/1
  I/1 -> Product1/2
  Product/1 -> Sum1/1
  Saturation1/1 -> Switch2/1
  err/1 -> Saturation1/1
  Constant1/1 -> Switch2/3
  reset/1 -> Logical Operator5/1, Switch3/2, Switch2/2
  Switch2/1 -> Unit Delay1/1, Sum2/1, Product1/1, Product/1
  P/1 -> Product/2
  Constant5/1 -> Switch4/3

== system PMSM20180521/Subsystem1/RC filter9 ==
  x : Inport
  Constant2 : Constant  Value=a  OutDataTypeStr=double
  Constant3 : Constant  Value=1-a  OutDataTypeStr=double
  Divide : Product
  Divide1 : Product
  Sum2 : Sum
  Unit Delay2 : UnitDelay  SampleTime=-1
  y : Outport
  wires:
  Unit Delay2/1 -> Divide1/2
  Sum2/1 -> Unit Delay2/1, y/1
  Divide1/1 -> Sum2/2
  Divide/1 -> Sum2/1
  Constant3/1 -> Divide1/1
  Constant2/1 -> Divide/2
  x/1 -> Divide/1

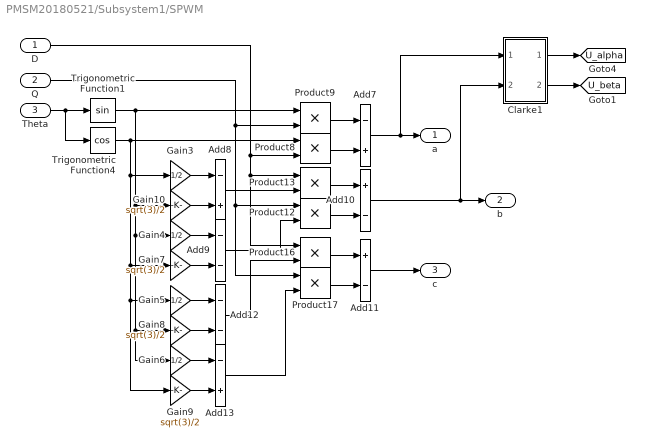
== system PMSM20180521/Subsystem1/SPWM ==
  D : Inport
  Q : Inport  Port=2
  Theta : Inport  Port=3
  Add10 : Sum  Inputs=+-
  Add11 : Sum  Inputs=+-
  Add12 : Sum  Inputs=--
  Add13 : Sum  Inputs=-+
  Add7 : Sum  Inputs=-+
  Add8 : Sum  Inputs=-+
  Add9 : Sum  Inputs=--
  Clarke1 : Subsystem
  Gain{7..10} (4 alike) : Gain  Gain=sqrt(3)/2
  Gain{3..6} (4 alike) : Gain  Gain=1/2
  Product{8..9,12..13,16..17} (6 alike) : Product  RndMeth=Zero
  Trigonometric Function1 : Trigonometry
  Trigonometric Function4 : Trigonometry  Operator=cos
  a : Outport
  b : Outport  Port=2
  c : Outport  Port=3
  tag scope: U_alpha=global, U_beta=global
  wires:
  Theta/1 -> Trigonometric Function1/1, Trigonometric Function4/1
  Trigonometric Function4/1 -> Product8/1, Gain3/1, Gain5/1, Gain9/1, Gain7/1
  Product8/1 -> Add7/2
  Trigonometric Function1/1 -> Product9/1, Gain4/1, Gain6/1, Gain8/1, Gain10/1
  Product9/1 -> Add7/1
  Gain3/1 -> Add8/1
  Gain4/1 -> Add9/1
  Gain7/1 -> Add9/2
  Product13/1 -> Add10/1
  Product12/1 -> Add10/2
  Add8/1 -> Product13/2
  Add9/1 -> Product12/2
  Product16/1 -> Add11/1
  Product17/1 -> Add11/2
  Add12/1 -> Product16/2
  Add13/1 -> Product17/2
  Add7/1 -> a/1, Clarke1/1(In1)
  Add10/1 -> b/1, Clarke1/2(In2)
  Add11/1 -> c/1
  Gain6/1 -> Add13/1
  Gain8/1 -> Add12/2
  Gain5/1 -> Add12/1
  Gain9/1 -> Add13/2
  Gain10/1 -> Add8/2
  D/1 -> Product8/2, Product13/1, Product16/1
  Q/1 -> Product9/2, Product12/1, Product17/1
  Clarke1/1(alpha) -> [U_alpha]
  Clarke1/2(beta) -> [U_beta]

== system PMSM20180521/Subsystem1/Subsystem2 ==
  In1 : Inport
  In2 : Inport  Port=2
  Product : Product  RndMeth=Zero
  Product1 : Product  RndMeth=Zero
  Sqrt : Sqrt  SaturateOnIntegerOverflow=on
  Sum17 : Sum
  Out1 : Outport
  wires:
  Product/1 -> Sum17/1
  Product1/1 -> Sum17/2
  Sum17/1 -> Sqrt/1
  In1/1 -> Product/2, Product/1
  In2/1 -> Product1/2, Product1/1
  Sqrt/1 -> Out1/1

== system PMSM20180521/Subsystem1/abc/dq current ==
  iga : Inport
  igb : Inport  Port=2
  angle : Inport  Port=3
  Clarke1 : Subsystem
  Park1 : Subsystem
  igd : Outport
  igq : Outport  Port=2
  tag scope: i_alpha=global, i_beta=global
  wires:
  Park1/1(d) -> igd/1
  iga/1 -> Clarke1/1(In1)
  Park1/2(q) -> igq/1
  igb/1 -> Clarke1/2(In2)
  Clarke1/1(alpha) -> Park1/1(alpha), [i_alpha]
  Clarke1/2(beta) -> Park1/2(beta), [i_beta]
  angle/1 -> Park1/3(theta)

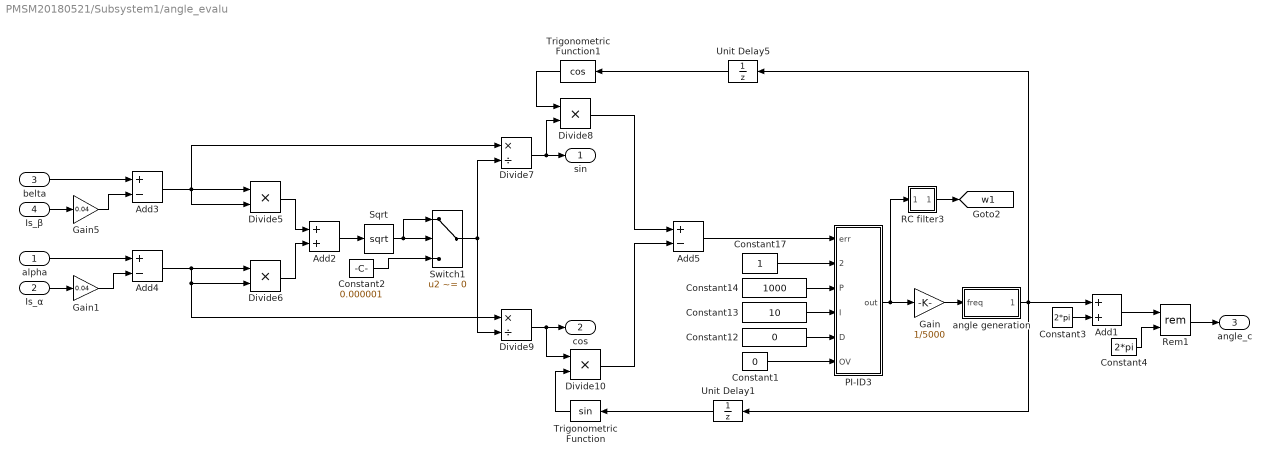
== system PMSM20180521/Subsystem1/angle_evalu ==
  alpha : Inport
  Is_α : Inport  Port=2
  belta : Inport  Port=3
  Is_β : Inport  Port=4
  Add1 : Sum
  Add2 : Sum
  Add3 : Sum  Inputs=+-
  Add4 : Sum  Inputs=+-
  Add5 : Sum  Inputs=+-
  Constant1 : Constant  Value=0  OutDataTypeStr=double
  Constant12 : Constant  Value=0  OutDataTypeStr=double
  Constant13 : Constant  Value=10  OutDataTypeStr=double
  Constant14 : Constant  Value=1000  OutDataTypeStr=double
  Constant17 : Constant  OutDataTypeStr=double
  Constant2 : Constant  Value=0.000001  OutDataTypeStr=double
  Constant3 : Constant  Value=2*pi  OutDataTypeStr=double
  Constant4 : Constant  Value=2*pi  OutDataTypeStr=double
  Divide{5..6,8,10} (4 alike) : Product  Inputs=**
  Divide7 : Product  Inputs=*/
  Divide9 : Product  Inputs=*/
  Gain : Gain  Gain=1/5000
  Gain1 : Gain  Gain=0.04
  Gain5 : Gain  Gain=0.04
  PI-ID3 : Subsystem  mask{ermax=0.5*pi, ermin=-0.5*pi, max=500, min=-500}
      mask prompts: ermax "Err max limit"; ermin "Err min limit"; max "Output max limit"; min "Output min limit"
  RC filter3 : Subsystem  mask{a=0.8}
      mask prompts: a "Time Constant"
  Rem1 : Math  Operator=rem  SaturateOnIntegerOverflow=on
  Sqrt : Sqrt  SaturateOnIntegerOverflow=on
  Switch1 : Switch  Criteria=u2 ~= 0
  Trigonometric Function : Trigonometry
  Trigonometric Function1 : Trigonometry  Operator=cos
  Unit Delay1 : UnitDelay  SampleTime=-1
  Unit Delay5 : UnitDelay  SampleTime=-1
  angle generation : Subsystem
  sin : Outport
  cos : Outport  Port=2
  angle_c : Outport  Port=3
  tag scope: w1=global
  wires:
  belta/1 -> Add3/1
  Add3/1 -> Divide5/1, Divide5/2, Divide7/1
  Gain5/1 -> Add3/2
  Gain1/1 -> Add4/2
  Is_β/1 -> Gain5/1
  Is_α/1 -> Gain1/1
  Add4/1 -> Divide6/1, Divide6/2, Divide9/1
  Divide5/1 -> Add2/1
  Divide6/1 -> Add2/2
  Add2/1 -> Sqrt/1
  Divide7/1 -> sin/1, Divide8/2
  Divide9/1 -> cos/1, Divide10/1
  Trigonometric Function/1 -> Divide10/2
  Divide8/1 -> Add5/1
  Divide10/1 -> Add5/2
  Add5/1 -> PI-ID3/1(err)
  Constant17/1 -> PI-ID3/2(reset)
  Constant12/1 -> PI-ID3/5(D)
  Constant1/1 -> PI-ID3/6(OV)
  Constant14/1 -> PI-ID3/3(P)
  Constant13/1 -> PI-ID3/4(I)
  Gain/1 -> angle generation/1(freq)
  PI-ID3/1(out) -> Gain/1, RC filter3/1(x)
  angle generation/1(angle_0) -> Unit Delay5/1, Unit Delay1/1, Add1/1
  Unit Delay5/1 -> Trigonometric Function1/1
  Unit Delay1/1 -> Trigonometric Function/1
  Trigonometric Function1/1 -> Divide8/1
  Sqrt/1 -> Switch1/2, Switch1/1
  Constant2/1 -> Switch1/3
  Switch1/1 -> Divide7/2, Divide9/2
  RC filter3/1(y) -> [w1]
  alpha/1 -> Add4/1
  Constant3/1 -> Add1/2
  Constant4/1 -> Rem1/2
  Add1/1 -> Rem1/1
  Rem1/1 -> angle_c/1

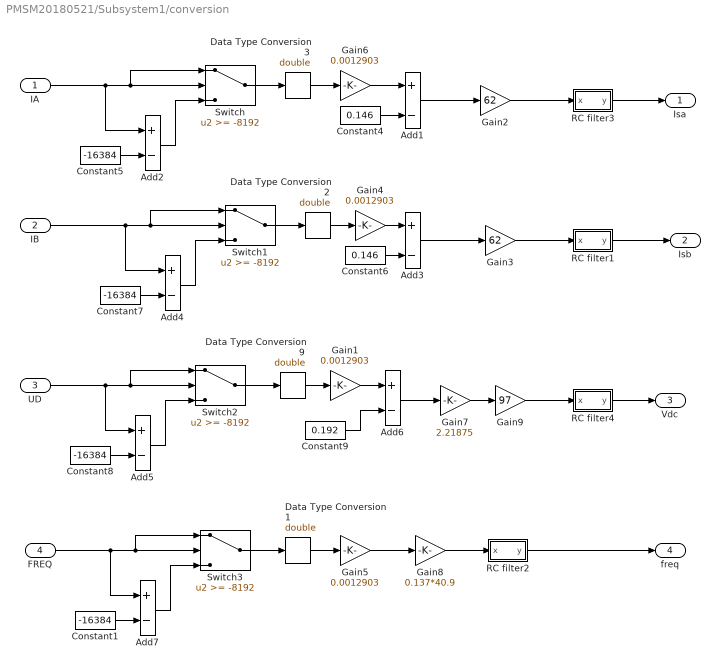
== system PMSM20180521/Subsystem1/conversion ==
  IA : Inport
  IB : Inport  Port=2
  UD : Inport  Port=3
  FREQ : Inport  Port=4
  Add{1..7} (7 alike) : Sum  Inputs=+-
  Constant{1,5,7..8} (4 alike) : Constant  Value=-16384  OutDataTypeStr=int16
  Constant4 : Constant  Value=0.146  OutDataTypeStr=double
  Constant6 : Constant  Value=0.146  OutDataTypeStr=double
  Constant9 : Constant  Value=0.192  OutDataTypeStr=double
  Data Type Conversion{1..3,9} (4 alike) : DataTypeConversion  OutDataTypeStr=double
  Gain{1,4..6} (4 alike) : Gain  Gain=0.0012903
  Gain2 : Gain  Gain=62
  Gain3 : Gain  Gain=62
  Gain7 : Gain  Gain=2.21875
  Gain8 : Gain  Gain=0.137*40.9
  Gain9 : Gain  Gain=97
  RC filter1 : Subsystem  mask{a=0.5}
      mask prompts: a "Time Constant"
  RC filter2 : Subsystem  mask{a=0.1}
      mask prompts: a "Time Constant"
  RC filter3 : Subsystem  mask{a=0.5}
      mask prompts: a "Time Constant"
  RC filter4 : Subsystem  mask{a=0.1}
      mask prompts: a "Time Constant"
  Switch{,1..3} (4 alike) : Switch  Threshold=-8192
  Isa : Outport
  Isb : Outport  Port=2
  Vdc : Outport  Port=3
  freq : Outport  Port=4
  wires:
  UD/1 -> Switch2/1, Switch2/2, Add5/1
  IA/1 -> Switch/1, Switch/2, Add2/1
  Constant5/1 -> Add2/2
  Add2/1 -> Switch/3
  Switch/1 -> Data Type Conversion3/1
  Data Type Conversion3/1 -> Gain6/1
  Gain2/1 -> RC filter3/1(x)
  Add1/1 -> Gain2/1
  Gain6/1 -> Add1/1
  Constant4/1 -> Add1/2
  IB/1 -> Switch1/1, Switch1/2, Add4/1
  Constant7/1 -> Add4/2
  Add4/1 -> Switch1/3
  Switch1/1 -> Data Type Conversion2/1
  Data Type Conversion2/1 -> Gain4/1
  Add3/1 -> Gain3/1
  Gain4/1 -> Add3/1
  Constant6/1 -> Add3/2
  Data Type Conversion9/1 -> Gain1/1
  Gain7/1 -> Gain9/1
  Constant8/1 -> Add5/2
  Add5/1 -> Switch2/3
  Switch2/1 -> Data Type Conversion9/1
  Gain1/1 -> Add6/1
  Add6/1 -> Gain7/1
  Constant9/1 -> Add6/2
  FREQ/1 -> Switch3/1, Switch3/2, Add7/1
  Data Type Conversion1/1 -> Gain5/1
  Constant1/1 -> Add7/2
  Add7/1 -> Switch3/3
  Switch3/1 -> Data Type Conversion1/1
  Gain5/1 -> Gain8/1
  RC filter2/1(y) -> freq/1
  Gain8/1 -> RC filter2/1(x)
  RC filter1/1(y) -> Isb/1
  RC filter3/1(y) -> Isa/1
  RC filter4/1(y) -> Vdc/1
  Gain9/1 -> RC filter4/1(x)
  Gain3/1 -> RC filter1/1(x)
